simulink model "lander0102no1"  (R2019b)
settings: Solver=VariableStepAuto  StartTime=0.0  StopTime=150  RelTol=1e-3
model workspace (MAT data in the model file):
  R = 1738000
  myu = 4903000000000
libraries: simulink_extras x6
settings Model: Creator=hp731  LastModifiedBy=hp731

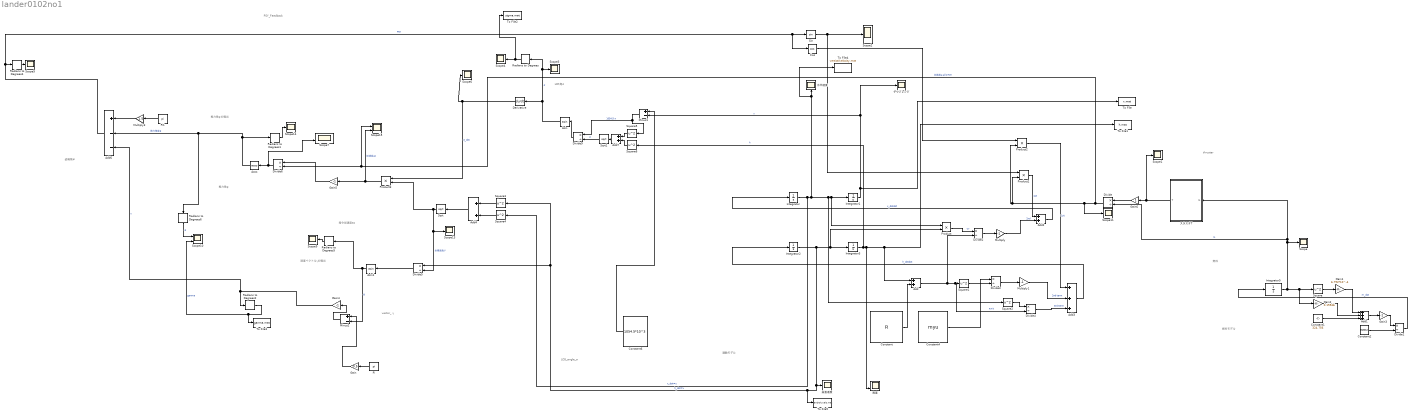
== system lander0102no1 ==
  note: thruster
  note: LOS_angle_σ
  note: 姿勢角Ψ
  note: LOS角σ
  note: 燃料
  note: 指令加速度ac
  note: vector_ γ
  note: 推力角φ
  note: 運動モデル
  note: 速度ベクトルγの導出
  note: 推力角φの導出
  note: 燃料モデル
  note: PSY_Feedback
  Acos : Trigonometry  Operator=acos
  Add{,2,4,7} (4 alike) : Sum
  Add1 : Sum  Inputs=+++
  Add3 : Sum  Inputs=+++
  Add6 : Sum  Inputs=+--
  Asin : Trigonometry  Operator=asin
  Asin1 : Trigonometry  Operator=asin
  Constant : Constant  Value=R
  Constant1 : Constant  Value=324.756
  Constant2 : Constant  Value=3138.2
  Constant4 : Constant  Value=myu
  Constant6 : Constant  Value=1054.5*10^3
  Cos : Trigonometry  Operator=cos
  Derivative : Derivative  CoefficientInTFapproximation=1
  Divide{,2..4,6} (5 alike) : Product  Inputs=*/  SaturateOnIntegerOverflow=on  RndMeth=Zero
  Divide1 : Product  Inputs=*/
  Divide5 : Product  Inputs=*/
  Divide9 : Product  Inputs=*/
  Gain : Gain  Gain=0.5
  Gain1 : Gain  Gain=6.792*10^-4
  Gain2 : Gain  Gain=0.15946
  Gain3 : Gain  Gain=-1
  Gain4 : Gain  Gain=-1
  Gain5 : Gain  Gain=-1
  Gain6 : Gain
  Integrator : Integrator  InitialCondition=170
  Integrator1 : Integrator  InitialCondition=1040.7*10^3
  Integrator2 : Integrator  InitialCondition=3
  Integrator3 : Integrator  InitialCondition=0.5*10^3
  Integrator5 : Integrator  InitialCondition=165.33
  Minus1 : Sum  Inputs=+-
  Minus2 : Sum  Inputs=+-
  Multiply : Gain  Gain=-1
  Multiply1 : Gain  Gain=-1
  Multiply3 : Gain  Gain=1.5
  Pi : Constant  Value=pi  OutDataTypeStr=Inherit: Inherit via back propagation
  Pi1 : Constant  Value=pi  OutDataTypeStr=Inherit: Inherit via back propagation
  Product{,1..3} (4 alike) : Product
  Radians to Degrees{,1..2,4..6} (6 alike) : simulink_extras/Transformations/Radians to Degrees
  Scope{,1..6,9,11,13..14} (11 alike) : Scope
  Scope10 : Scope  NumInputPorts=2
  Scope15 : Scope  NumInputPorts=2
  Scope7 : Scope  NumInputPorts=2
  Sin : Trigonometry
  Sqrt : Sqrt  SaturateOnIntegerOverflow=on
  Sqrt1 : Sqrt  SaturateOnIntegerOverflow=on
  Square{,1..4} (5 alike) : Math  Operator=square  SaturateOnIntegerOverflow=on
  Square5 : Math  Operator=square  SignedPower=off  SaturateOnIntegerOverflow=on
  Square6 : Math  Operator=square  SignedPower=off  SaturateOnIntegerOverflow=on
  To File : ToFile  Filename=x.mat  SaveFormat=Timeseries
  To File1 : ToFile  Filename=h.mat  SaveFormat=Timeseries
  To File2 : ToFile  Filename=sigma.mat  SaveFormat=Timeseries
  To File3 : ToFile  Filename=ganma.mat  SaveFormat=Timeseries
  To File4 : ToFile  Filename=verticalvelocity.mat  SaveFormat=Timeseries
  To File5 : ToFile  Filename=enchokuvelo.mat  SaveFormat=Timeseries
  スラスタT : Subsystem
  ダウンレンジ : Scope
  水平速度 : Scope
  鉛直速度 : Scope
  高度 : Scope  NumInputPorts=2
  wires:
  スラスタT/1(T) -> Gain6/1, Scope1/1
  Constant/1 -> Add/2
  Multiply3/1 -> Add6/1
  Constant2/1 -> Divide1/2
  Square3/1 -> Add4/1
  Asin/1 -> Derivative/1, Scope3/1, Radians to Degrees/1  "σ"
  Divide6/1 -> Scope7/2, Acos/1
  Product1/1 -> Add2/1  "1st"
  Gain4/1 -> Add6/3, Radians to Degrees2/1  "γ"
  Square2/1 -> Divide4/1
  Add4/1 -> Sqrt/1
  Radians to Degrees/1 -> To File2/1, Scope4/1
  Divide4/1 -> Add3/3  "3rd term"
  Constant6/1 -> Minus1/1
  Pi1/1 -> Multiply3/1
  Add/1 -> Divide4/2, Square1/1, Divide2/2  "R+h"
  Acos/1 -> Add6/2, Radians to Degrees6/1, Radians to Degrees1/1  "推力角度φ"
  Integrator/1 -> Square4/1, To File4/1, 水平速度/1, Square2/1, Product/1, Integrator1/1  "x_dot=u"
  Asin1/1 -> Minus2/2, Radians to Degrees5/1  "θ"
  Multiply/1 -> Add2/2  "2nd"
  Product3/1 -> Gain5/1, Scope15/2  "加速度ac"
  Product2/1 -> Add3/1  "1st"
  Add3/1 -> Integrator2/1  "h_dotdot"
  Minus1/1 -> Divide9/1, Square5/1  "1054.5-x"
  Integrator2/1 -> To File5/1, Divide5/1, Square3/1, 鉛直速度/1, Product/2, Integrator3/1  "h_dot=v"
  Sqrt/1 -> Product3/2, Divide5/2, Scope13/1  "全機速度V"
  Cos/1 -> Product2/1
  Sin/1 -> Product1/1, Scope2/1
  Divide2/1 -> Multiply/1
  Add2/1 -> Integrator/1  "x_dotdot"
  Integrator1/1 -> To File/1, ダウンレンジ/1, Minus1/2  "x"
  Multiply1/1 -> Add3/2  "2nd term"
  Divide3/1 -> Multiply1/1
  Integrator3/1 -> Square6/1, 高度/2, To File1/1, Add/1  "h"
  Constant4/1 -> Divide3/1
  Add1/1 -> Gain3/1
  Gain3/1 -> Divide1/1
  Gain2/1 -> Add1/2
  Constant1/1 -> Add1/3
  Divide1/1 -> Integrator5/1  "m_dot"
  Gain1/1 -> Add1/1
  Square4/1 -> Add4/2
  Divide/1 -> Scope15/1, Divide6/2, Scope11/1, Product2/2, Product1/2  "加速度a all=T/m"
  Integrator5/1 -> Divide/2, スラスタT/1(m), Scope/1, Gain2/1, Square/1  "m"
  Square/1 -> Gain1/1
  Square1/1 -> Divide3/2
  Product/1 -> Divide2/1  "uv"
  Add6/1 -> Cos/1, Sin/1, Radians to Degrees4/1  "PSY"
  Square5/1 -> Add7/1
  Square6/1 -> Add7/2
  Add7/1 -> Sqrt1/1
  Sqrt1/1 -> Divide9/2  "ρ"
  Divide9/1 -> Asin/1
  Divide5/1 -> Asin1/1
  Radians to Degrees4/1 -> Scope5/1
  Radians to Degrees2/1 -> Scope10/2, To File3/1  "ganma"
  Radians to Degrees5/1 -> Scope9/1
  Pi/1 -> Gain/1
  Gain/1 -> Minus2/1
  Minus2/1 -> Gain4/1
  Radians to Degrees6/1 -> Scope10/1  "Φ"
  Radians to Degrees1/1 -> Scope14/1
  Derivative/1 -> Product3/1, Scope6/1  "σ_dot"
  Gain5/1 -> Divide6/1
  Gain6/1 -> Divide/1

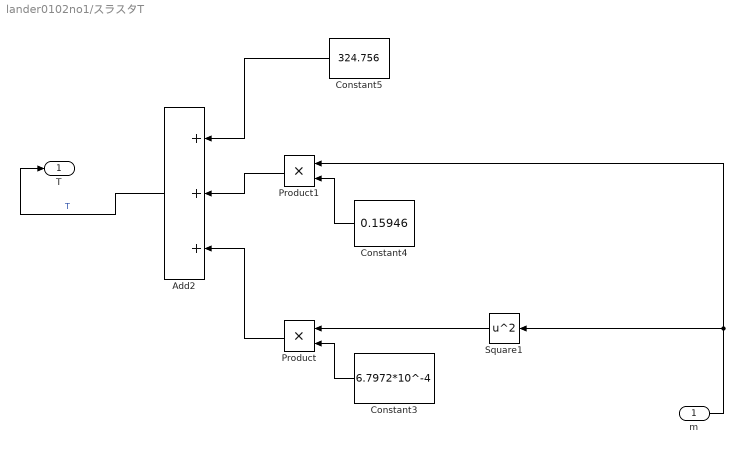
== system lander0102no1/スラスタT ==
  m : Inport
  Add2 : Sum  Inputs=+++
  Constant3 : Constant  Value=6.7972*10^-4
  Constant4 : Constant  Value=0.15946
  Constant5 : Constant  Value=324.756
  Product : Product
  Product1 : Product
  Square1 : Math  Operator=square  SaturateOnIntegerOverflow=on
  T : Outport  VectorParamsAs1DForOutWhenUnconnected=off
  wires:
  Product/1 -> Add2/3
  Constant3/1 -> Product/2
  Add2/1 -> T/1  "T"
  m/1 -> Product1/1, Square1/1
  Square1/1 -> Product/1
  Constant5/1 -> Add2/1
  Product1/1 -> Add2/2
  Constant4/1 -> Product1/2
